simulink model "DT4V_System_Model_v17_ref_speed_R2019a"  (R2023a)
settings: Solver=ode4  StartTime=0.0  StopTime=Config.Tsim  FixedStep=Config.Ts  RelTol=1e-3
undefined symbols (not defined in the file or in its folder): CC, Config, DCL, DiscIntNeverNeededParam, EM, GB, Grid, Inv, LM, Ma_1D, Psw_1D, Rceon_1D, Rec, Vceon_1D
libraries: simulink x3, DT4V_LoadModels x2
(part 2 of 2)

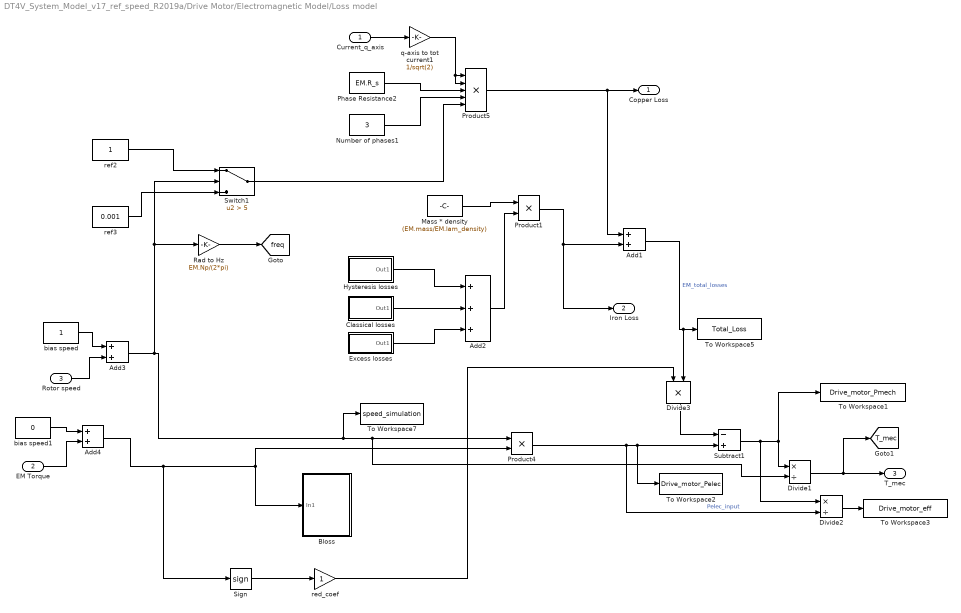
== system DT4V_System_Model_v17_ref_speed_R2019a/Drive Motor/Electromagnetic Model/Loss model ==
  Current_q_axis : Inport
  EM Torque : Inport  Port=2
  Rotor speed : Inport  Port=3
  Add1 : Sum
  Add2 : Sum  Inputs=+++
  Add3 : Sum
  Add4 : Sum
  Bloss : Subsystem
  Classical losses : Subsystem
  Divide1 : Product  Inputs=*/
  Divide2 : Product  Inputs=*/
  Divide3 : Product  Inputs=**
  Excess losses : Subsystem
  Hysteresis losses : Subsystem
  Mass * density : Constant  Value=(EM.mass/EM.lam_density)
  Number of phases1 : Constant  Value=3
  Phase Resistance2 : Constant  Value=EM.R_s
  Product1 : Product
  Product4 : Product
  Product5 : Product  Inputs=5
  Rad to Hz : Gain  Gain=EM.Np/(2*pi)
  Sign : Signum
  Subtract1 : Sum  Inputs=-+
  Switch1 : Switch  Criteria=u2 > Threshold  Threshold=5  SaturateOnIntegerOverflow=off  InputSameDT=off
  To Workspace1 : ToWorkspace  VariableName=Drive_motor_Pmech  SampleTime=-1
      settings: Save2DSignal=2-D array (concatenate along first dimension)
  To Workspace2 : ToWorkspace  VariableName=Drive_motor_Pelec  SampleTime=-1
      settings: Save2DSignal=2-D array (concatenate along first dimension)
  To Workspace3 : ToWorkspace  VariableName=Drive_motor_eff  SampleTime=-1
      settings: Save2DSignal=2-D array (concatenate along first dimension)
  To Workspace5 : ToWorkspace  VariableName=Total_Loss  SampleTime=-1
      settings: Save2DSignal=2-D array (concatenate along first dimension)
  To Workspace7 : ToWorkspace  VariableName=speed_simulation  SampleTime=-1
      settings: Save2DSignal=2-D array (concatenate along first dimension)
  bias speed : Constant
  bias speed1 : Constant  Value=0
  q-axis to tot current1 : Gain  Gain=1/sqrt(2)
  red_coef : Gain
  ref2 : Constant
  ref3 : Constant  Value=0.001
  "Copper Loss " : Outport
  Iron Loss : Outport  Port=2
  T_mec : Outport  Port=3
  tag scope: T_mec=global, freq=global
  wires:
  Product1/1 -> Iron Loss/1, Add1/2
  Number of phases1/1 -> Product5/4
  Excess losses/1(Out1) -> Add2/3
  Hysteresis losses/1(Out1) -> Add2/1
  Rad to Hz/1 -> [freq]
  Add1/1 -> To Workspace5/1, Divide3/2  "EM_total_losses"
  Subtract1/1 -> Divide2/1, Divide1/1, To Workspace1/1
  Classical losses/1(Out1) -> Add2/2
  Current_q_axis/1 -> q-axis to tot current1/1
  Phase Resistance2/1 -> Product5/3
  Add3/1 -> To Workspace7/1, Product4/1, Divide1/2, Switch1/2, Rad to Hz/1
  Product4/1 -> Divide2/2, To Workspace2/1, Subtract1/2  "Pelec_input"
  q-axis to tot current1/1 -> Product5/2, Product5/1
  Add2/1 -> Product1/2
  ref3/1 -> Switch1/3
  ref2/1 -> Switch1/1
  Divide2/1 -> To Workspace3/1
  Divide1/1 -> [T_mec], T_mec/1
  Add4/1 -> Sign/1, Product4/2, Bloss/1(In1)
  Sign/1 -> red_coef/1
  Product5/1 -> "Copper Loss "/1, Add1/1
  Divide3/1 -> Subtract1/1
  red_coef/1 -> Divide3/1
  bias speed/1 -> Add3/1
  Rotor speed/1 -> Add3/2
  Switch1/1 -> Product5/5
  bias speed1/1 -> Add4/1
  EM Torque/1 -> Add4/2
  Mass * density/1 -> Product1/1

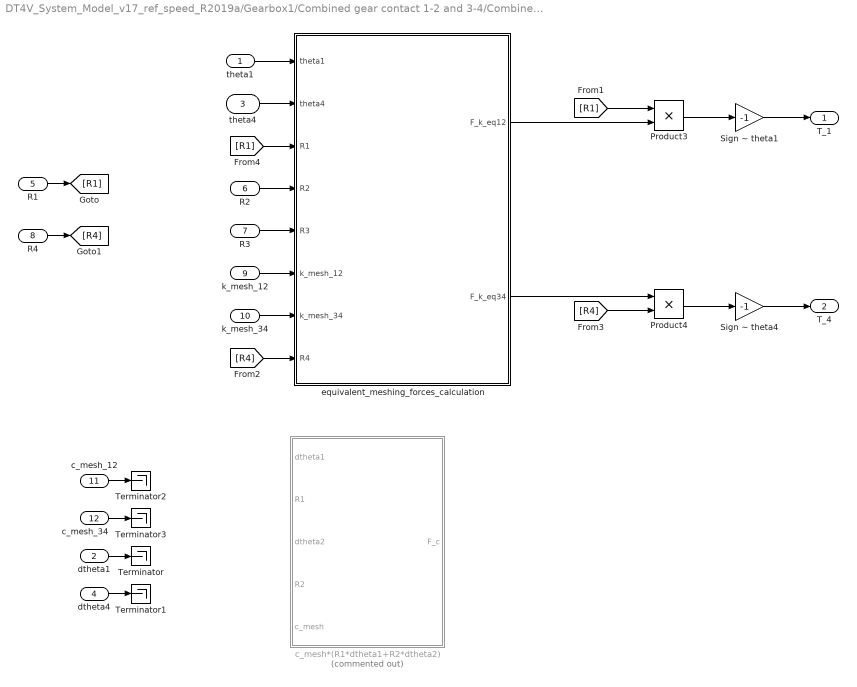
== system DT4V_System_Model_v17_ref_speed_R2019a/Gearbox1/Combined gear contact 1-2 and 3-4/Combined contact 1-2, 3-4 ==
  theta1 : Inport
  dtheta1 : Inport  Port=2
  theta4 : Inport  Port=3
  dtheta4 : Inport  Port=4
  R1 : Inport  Port=5
  R2 : Inport  Port=6
  R3 : Inport  Port=7
  R4 : Inport  Port=8
  k_mesh_12 : Inport  Port=9
  k_mesh_34 : Inport  Port=10
  c_mesh_12 : Inport  Port=11
  c_mesh_34 : Inport  Port=12
  Product3 : Product
  Product4 : Product
  Sign ~ theta1 : Gain  Gain=-1
  Sign ~ theta4 : Gain  Gain=-1
  Terminator{,1..3} (4 alike) : Terminator
  c_mesh*(R1*dtheta1+R2*dtheta2) : Subsystem  Commented=on
  equivalent_meshing_forces_calculation : Subsystem
  T_1 : Outport
  T_4 : Outport  Port=2
  wires:
  theta1/1 -> equivalent_meshing_forces_calculation/1(theta1)
  k_mesh_12/1 -> equivalent_meshing_forces_calculation/6(k_mesh_12)
  [R1] -> equivalent_meshing_forces_calculation/3(R1)
  [R1] -> Product3/1
  R2/1 -> equivalent_meshing_forces_calculation/4(R2)
  [R4] -> Product4/2
  equivalent_meshing_forces_calculation/1(F_k_eq12) -> Product3/2
  Product3/1 -> Sign ~ theta1/1
  Sign ~ theta1/1 -> T_1/1
  Product4/1 -> Sign ~ theta4/1
  Sign ~ theta4/1 -> T_4/1
  dtheta1/1 -> Terminator/1
  dtheta4/1 -> Terminator1/1
  c_mesh_12/1 -> Terminator2/1
  c_mesh_34/1 -> Terminator3/1
  theta4/1 -> equivalent_meshing_forces_calculation/2("theta4 ")
  R3/1 -> equivalent_meshing_forces_calculation/5(R3)
  k_mesh_34/1 -> equivalent_meshing_forces_calculation/7(k_mesh_34)
  R1/1 -> [R1]
  R4/1 -> [R4]
  [R4] -> equivalent_meshing_forces_calculation/8(R4)
  equivalent_meshing_forces_calculation/2(F_k_eq34) -> Product4/1

== system DT4V_System_Model_v17_ref_speed_R2019a/Gearbox1/Thermal model/Heat equation ==
  P_loss : Inport
  UA : Inport  Port=2
  T_ambient : Inport  Port=3
  -(T-T_env) : Sum  Inputs=-+
  1/(m*C_P) : Product  Inputs=*/
  Add : Sum  OutMin=[-1e6]  OutMax=[1e6]
  Constant1 : Constant
  Integrator : Integrator  InitialCondition=GB.oil.temp_0
  Product2 : Product
  dT_dt : Product
  mcp : Constant  Value=GB.thermal.mcpeq
  T : Outport
  wires:
  -(T-T_env)/1 -> Product2/2
  UA/1 -> Product2/1
  Product2/1 -> Add/2
  1/(m*C_P)/1 -> dT_dt/2
  Add/1 -> dT_dt/1
  Constant1/1 -> 1/(m*C_P)/1
  P_loss/1 -> Add/1
  T_ambient/1 -> -(T-T_env)/2
  dT_dt/1 -> Integrator/1
  Integrator/1 -> -(T-T_env)/1, T/1
  mcp/1 -> 1/(m*C_P)/2

== system DT4V_System_Model_v17_ref_speed_R2019a/Gearbox1/Zero inertia gear 1/Sign & maximum for loss term ==
  T_loss : Inport
  Speed : Inport  Port=2
  T_in : Inport  Port=3
  Abs1 : Abs  SaturateOnIntegerOverflow=off
  Abs2 : Abs  SaturateOnIntegerOverflow=off
  Gain1 : Gain  Gain=-1
  Gain2 : Gain  Gain=-1
  OR : Sum
  Relational Operator1 : RelationalOperator  Operator=<  OutDataTypeStr=boolean  RndMeth=Simplest  InputSameDT=off
  Should be positive (Just to be sure) : Abs  SaturateOnIntegerOverflow=off
  Sign loss torque : Switch  Criteria=u2 > Threshold  SaturateOnIntegerOverflow=off  InputSameDT=off
  Speed threshold : Constant  Value=0.001
  "Standard - loss opposite sign to speed Very low speed - loss opposite sign to torque " : Switch  Criteria=u2 > Threshold  SaturateOnIntegerOverflow=off  InputSameDT=off
  Very low speed Max. |T_loss| = |T_in| : Switch  Criteria=u2 > Threshold  SaturateOnIntegerOverflow=off  InputSameDT=off
  |T_loss| <= |T_in| : RelationalOperator  Operator=<=  OutDataTypeStr=boolean  RndMeth=Simplest  InputSameDT=off
  T_loss_correct_sign : Outport
  wires:
  T_in/1 -> "Standard - loss opposite sign to speed Very low speed - loss opposite sign to torque "/3, Abs1/1, Gain2/1
  Relational Operator1/1 -> "Standard - loss opposite sign to speed Very low speed - loss opposite sign to torque "/2, OR/2
  |T_loss| <= |T_in|/1 -> OR/1
  Should be positive (Just to be sure)/1 -> |T_loss| <= |T_in|/1, Sign loss torque/3, Gain1/1
  OR/1 -> Very low speed Max. |T_loss| = |T_in|/2
  Abs2/1 -> Relational Operator1/2
  Gain1/1 -> Sign loss torque/1
  Speed threshold/1 -> Relational Operator1/1
  Abs1/1 -> |T_loss| <= |T_in|/2
  Sign loss torque/1 -> Very low speed Max. |T_loss| = |T_in|/1
  Gain2/1 -> Very low speed Max. |T_loss| = |T_in|/3
  "Standard - loss opposite sign to speed Very low speed - loss opposite sign to torque "/1 -> Sign loss torque/2
  Speed/1 -> "Standard - loss opposite sign to speed Very low speed - loss opposite sign to torque "/1, Abs2/1
  Very low speed Max. |T_loss| = |T_in|/1 -> T_loss_correct_sign/1
  T_loss/1 -> Should be positive (Just to be sure)/1

== system DT4V_System_Model_v17_ref_speed_R2019a/Gearbox1/Zero inertia gear 4/Sign & maximum for loss term ==
  T_loss : Inport
  Speed : Inport  Port=2
  T_in : Inport  Port=3
  Abs1 : Abs  SaturateOnIntegerOverflow=off
  Abs2 : Abs  SaturateOnIntegerOverflow=off
  Gain1 : Gain  Gain=-1
  Gain2 : Gain  Gain=-1
  OR : Sum
  Relational Operator1 : RelationalOperator  Operator=<  OutDataTypeStr=boolean  RndMeth=Simplest  InputSameDT=off
  Should be positive (Just to be sure) : Abs  SaturateOnIntegerOverflow=off
  Sign loss torque : Switch  Criteria=u2 > Threshold  SaturateOnIntegerOverflow=off  InputSameDT=off
  Speed threshold : Constant  Value=0.001
  "Standard - loss opposite sign to speed Very low speed - loss opposite sign to torque " : Switch  Criteria=u2 > Threshold  SaturateOnIntegerOverflow=off  InputSameDT=off
  Very low speed Max. |T_loss| = |T_in| : Switch  Criteria=u2 > Threshold  SaturateOnIntegerOverflow=off  InputSameDT=off
  |T_loss| <= |T_in| : RelationalOperator  Operator=<=  OutDataTypeStr=boolean  RndMeth=Simplest  InputSameDT=off
  T_loss_correct_sign : Outport
  wires:
  T_in/1 -> "Standard - loss opposite sign to speed Very low speed - loss opposite sign to torque "/3, Abs1/1, Gain2/1
  Relational Operator1/1 -> "Standard - loss opposite sign to speed Very low speed - loss opposite sign to torque "/2, OR/2
  |T_loss| <= |T_in|/1 -> OR/1
  Should be positive (Just to be sure)/1 -> |T_loss| <= |T_in|/1, Sign loss torque/3, Gain1/1
  OR/1 -> Very low speed Max. |T_loss| = |T_in|/2
  Abs2/1 -> Relational Operator1/2
  Gain1/1 -> Sign loss torque/1
  Speed threshold/1 -> Relational Operator1/1
  Abs1/1 -> |T_loss| <= |T_in|/2
  Sign loss torque/1 -> Very low speed Max. |T_loss| = |T_in|/1
  Gain2/1 -> Very low speed Max. |T_loss| = |T_in|/3
  "Standard - loss opposite sign to speed Very low speed - loss opposite sign to torque "/1 -> Sign loss torque/2
  Speed/1 -> "Standard - loss opposite sign to speed Very low speed - loss opposite sign to torque "/1, Abs2/1
  Very low speed Max. |T_loss| = |T_in|/1 -> T_loss_correct_sign/1
  T_loss/1 -> Should be positive (Just to be sure)/1

== system DT4V_System_Model_v17_ref_speed_R2019a/Power Electronics2/AC//DC Converter/DC Bus model ==
  In1 : Inport
  1/C : Gain  Gain=1/(DCL.Cap.C_C_f)
  1/Rp : Gain  Gain=1/(DCL.Cap.Rp_C_ohm)
  Add : Sum  Inputs=+++
  Add1 : Sum  Inputs=-+
  Constant4 : Constant  Value=DCL.Cap.Vdc_C_v
  Integrator : Integrator  LimitOutput=on  UpperSaturationLimit=5  LowerSaturationLimit=-10  IgnoreLimit=on
  Memory : Memory
  Saturation : Saturate  UpperLimit=DCL.Cap.Vdcmax_C_v  LowerLimit=DCL.Cap.Vdcmin_C_v
  Transfer Fcn : TransferFcn  Denominator=[0.001 1]
  esr : Gain  Gain=DCL.Cap.ESR_C_ohm
  Voltage_DC_bus : Outport
  wires:
  In1/1 -> Transfer Fcn/1  "IDC_bus"
  Add/1 -> Saturation/1
  Constant4/1 -> Add/3
  Saturation/1 -> Voltage_DC_bus/1
  Add1/1 -> Memory/1, 1/C/1  "ic"
  1/C/1 -> Integrator/1
  Memory/1 -> 1/Rp/1
  Integrator/1 -> Add/1
  Transfer Fcn/1 -> Add1/2, esr/1
  esr/1 -> Add/2
  1/Rp/1 -> Add1/1

== system DT4V_System_Model_v17_ref_speed_R2019a/Power Electronics2/AC//DC Converter/Half-Bridge 1  ==
  Vdc : Inport
  Iphase : Inport  Port=2
  Constant4 : Constant  Value=Rec.Di.R0_3D_ohm
  Constant5 : Constant  Value=Rec.Di.VT_3D_v
  MATLAB Function : MATLAB Function  TreatAsAtomicUnit=on
  Vphase : Outport
  Idc : Outport  Port=2
  DiodeLosses1Phase : Outport  Port=3
  wires:
  Vdc/1 -> MATLAB Function/1(Vdc)
  MATLAB Function/2(Idc) -> Idc/1
  MATLAB Function/3(Pcond) -> DiodeLosses1Phase/1
  Iphase/1 -> MATLAB Function/2(Iphase)
  MATLAB Function/1(Vphase) -> Vphase/1
  Constant5/1 -> MATLAB Function/3(VT)
  Constant4/1 -> MATLAB Function/4(R_0)

== system DT4V_System_Model_v17_ref_speed_R2019a/Power Electronics2/AC//DC Converter/Half-Bridge 2 ==
  Vdc : Inport
  Iphase : Inport  Port=2
  Constant4 : Constant  Value=Rec.Di.R0_3D_ohm
  Constant5 : Constant  Value=Rec.Di.VT_3D_v
  MATLAB Function : MATLAB Function  TreatAsAtomicUnit=on
  Vphase : Outport
  Idc : Outport  Port=2
  DiodeLosses1Phase : Outport  Port=3
  wires:
  Vdc/1 -> MATLAB Function/1(Vdc)
  Iphase/1 -> MATLAB Function/2(Iphase)
  MATLAB Function/3(Pcond) -> DiodeLosses1Phase/1
  MATLAB Function/1(Vphase) -> Vphase/1
  MATLAB Function/2(Idc) -> Idc/1
  Constant4/1 -> MATLAB Function/4(R_0)
  Constant5/1 -> MATLAB Function/3(VT)

== system DT4V_System_Model_v17_ref_speed_R2019a/Power Electronics2/AC//DC Converter/Half-Bridge 3 ==
  Vdc : Inport
  Iphase : Inport  Port=2
  Constant4 : Constant  Value=Rec.Di.R0_3D_ohm
  Constant5 : Constant  Value=Rec.Di.VT_3D_v
  MATLAB Function : MATLAB Function  TreatAsAtomicUnit=on
  Vphase : Outport
  Idc : Outport  Port=2
  DiodeLosses1Phase : Outport  Port=3
  wires:
  Vdc/1 -> MATLAB Function/1(Vdc)
  Iphase/1 -> MATLAB Function/2(Iphase)
  MATLAB Function/3(Pcond) -> DiodeLosses1Phase/1
  MATLAB Function/1(Vphase) -> Vphase/1
  MATLAB Function/2(Idc) -> Idc/1
  Constant4/1 -> MATLAB Function/4(R_0)
  Constant5/1 -> MATLAB Function/3(VT)

== system DT4V_System_Model_v17_ref_speed_R2019a/Power Electronics2/AC//DC Converter/OverVoltage Control Block ==
  Enable/Disable : Inport
  Idc : Inport  Port=2
  AND : Logic  AllPortsSameDT=off  OutDataTypeStr=boolean
  Compare To Constant10 : simulink/Logic and Bit Operations/Compare To Constant  relop=<=  const=1  OutDataTypeStr=boolean
  Constant : Constant  Value=0
  Constant1 : Constant  Value=10
  Initial condition : Switch  Criteria=u2 > Threshold  SaturateOnIntegerOverflow=off  InputSameDT=off
  Memory : Memory
  Moving RMS Calculation Triggered Subsystem : Subsystem  TreatAsAtomicUnit=on
  Pulse Generator2 : DiscretePulseGenerator  PulseType=Time based  Period=Config.MovingRMS.Time  PulseWidth=((Config.MovingRMS.Time-Config.Ts)/(Config.MovingRMS.Time))*100  VectorParams1D=off
  Rate Transition : RateTransition  Deterministic=off  OutPortSampleTimeMultiple=Config.MovingRMS.Time  OutPortSampleTime=Config.MovingRMS.Time
  Step : Step  Time=Config.MovingRMS.Time  Before=1  After=0  SampleTime=0
  Switch : Switch  Criteria=u2 > Threshold  SaturateOnIntegerOverflow=off  InputSameDT=off
  Out1 : Outport
  wires:
  Switch/1 -> Out1/1
  AND/1 -> Switch/2
  Idc/1 -> Switch/3, Moving RMS Calculation Triggered Subsystem/1(In1)
  Pulse Generator2/1 -> Moving RMS Calculation Triggered Subsystem/Enable
  Constant/1 -> Switch/1
  Moving RMS Calculation Triggered Subsystem/1(Out1) -> Memory/1
  Step/1 -> Initial condition/2
  Rate Transition/1 -> Initial condition/3
  Constant1/1 -> Initial condition/1
  Memory/1 -> Rate Transition/1
  Initial condition/1 -> Compare To Constant10/1
  Enable/Disable/1 -> AND/2
  Compare To Constant10/1 -> AND/1

== system DT4V_System_Model_v17_ref_speed_R2019a/Power Electronics2/DC//AC Converter/AC Ouput power measurment ==
  Current : Inport
  Voltage : Inport  Port=2
  Product1 : Product  InputSameDT=on  SaturateOnIntegerOverflow=on  OutDataTypeStr=Inherit: Same as first input
  Sum4 : Sum  Inputs=1  InputSameDT=on  SaturateOnIntegerOverflow=on  OutDataTypeStr=Inherit: Same as first input
  Transfer Fcn1 : TransferFcn  Denominator=[0.005 1]
  AC ouput power : Outport
  wires:
  Voltage/1 -> Product1/2
  Current/1 -> Product1/1
  Product1/1 -> Sum4/1
  Sum4/1 -> Transfer Fcn1/1  "P"
  Transfer Fcn1/1 -> AC ouput power/1

== system DT4V_System_Model_v17_ref_speed_R2019a/Power Electronics2/DC//AC Converter/DC Input power measurment ==
  Current : Inport
  Voltage : Inport  Port=2
  Product1 : Product  InputSameDT=on  SaturateOnIntegerOverflow=on  OutDataTypeStr=Inherit: Same as first input
  Transfer Fcn1 : TransferFcn  Denominator=[0.005 1]
  DC input power : Outport
  wires:
  Product1/1 -> Transfer Fcn1/1  "P"
  Current/1 -> Product1/1
  Voltage/1 -> Product1/2
  Transfer Fcn1/1 -> DC input power/1

== system DT4V_System_Model_v17_ref_speed_R2019a/Power Electronics2/DC//AC Converter/Half-Bridge 1 ==
  d : Inport
  Vdc : Inport  Port=2
  Iphase : Inport  Port=3
  Constant2 : Constant  Value=Inv.IGBT.Rce_3D_ohm
  Constant3 : Constant  Value=Inv.IGBT.Vce_3D_v
  Constant4 : Constant  Value=Inv.Di.Rd_3D_ohm
  Constant5 : Constant  Value=Inv.Di.Vf_3D_v
  MATLAB Function : MATLAB Function  TreatAsAtomicUnit=on
  Vphase : Outport
  Idc : Outport  Port=2
  tag scope: P_cond_1=global
  wires:
  d/1 -> MATLAB Function/1(d)
  Vdc/1 -> MATLAB Function/2(Vdc)
  Iphase/1 -> MATLAB Function/3(Iphase)
  Constant2/1 -> MATLAB Function/5(Rce_on)
  Constant4/1 -> MATLAB Function/7(Rd)
  Constant3/1 -> MATLAB Function/4(Vce_on)
  Constant5/1 -> MATLAB Function/6(Vf_0)
  MATLAB Function/1(Vphase) -> Vphase/1
  MATLAB Function/2(Idc) -> Idc/1
  MATLAB Function/3(Pcond) -> [P_cond_1]

== system DT4V_System_Model_v17_ref_speed_R2019a/Power Electronics2/DC//AC Converter/Half-Bridge 2 ==
  d : Inport
  Vdc : Inport  Port=2
  Iphase : Inport  Port=3
  Constant2 : Constant  Value=Inv.IGBT.Rce_3D_ohm
  Constant3 : Constant  Value=Inv.IGBT.Vce_3D_v
  Constant4 : Constant  Value=Inv.Di.Rd_3D_ohm
  Constant5 : Constant  Value=Inv.Di.Vf_3D_v
  MATLAB Function : MATLAB Function  TreatAsAtomicUnit=on
  Vphase : Outport
  Idc : Outport  Port=2
  tag scope: P_cond_2=global
  wires:
  MATLAB Function/3(Pcond) -> [P_cond_2]
  MATLAB Function/1(Vphase) -> Vphase/1
  d/1 -> MATLAB Function/1(d)
  Iphase/1 -> MATLAB Function/3(Iphase)
  Constant4/1 -> MATLAB Function/7(Rd)
  Constant3/1 -> MATLAB Function/4(Vce_on)
  Constant2/1 -> MATLAB Function/5(Rce_on)
  Vdc/1 -> MATLAB Function/2(Vdc)
  Constant5/1 -> MATLAB Function/6(Vf_0)
  MATLAB Function/2(Idc) -> Idc/1

== system DT4V_System_Model_v17_ref_speed_R2019a/Power Electronics2/DC//AC Converter/Half-Bridge 3 ==
  d : Inport
  Vdc : Inport  Port=2
  Iphase : Inport  Port=3
  Constant2 : Constant  Value=Inv.IGBT.Rce_3D_ohm
  Constant3 : Constant  Value=Inv.IGBT.Vce_3D_v
  Constant4 : Constant  Value=Inv.Di.Rd_3D_ohm
  Constant5 : Constant  Value=Inv.Di.Vf_3D_v
  MATLAB Function : MATLAB Function  TreatAsAtomicUnit=on
  Vphase : Outport
  Idc : Outport  Port=2
  tag scope: P_cond_3=global
  wires:
  MATLAB Function/3(Pcond) -> [P_cond_3]
  MATLAB Function/1(Vphase) -> Vphase/1
  d/1 -> MATLAB Function/1(d)
  Iphase/1 -> MATLAB Function/3(Iphase)
  Constant4/1 -> MATLAB Function/7(Rd)
  Constant3/1 -> MATLAB Function/4(Vce_on)
  Constant2/1 -> MATLAB Function/5(Rce_on)
  Vdc/1 -> MATLAB Function/2(Vdc)
  Constant5/1 -> MATLAB Function/6(Vf_0)
  MATLAB Function/2(Idc) -> Idc/1

== system DT4V_System_Model_v17_ref_speed_R2019a/Power Electronics2/DC//AC Converter/Loss Model ==
  speed : Inport
  Torque : Inport  Port=2
  Power_Loss_Model1 : Subsystem  mask{sfcnParam1=Ma_1D, sfcnParam2=Psw_1D, sfcnParam3=Rceon_1D, sfcnParam4=Vceon_1D}
      mask prompts: sfcnParam1 "Ma_1D:"; sfcnParam2 "Psw_1D:"; sfcnParam3 "Rceon_1D:"; sfcnParam4 "Vceon_1D:"
      mask help: Simulink:masks:GenSFuncDesc_MD
      mask Help: eval('feval(''rtwprivate'',''rtwhelpview'',''rtw_sfcn_block'')');
  Sum3 : Sum  Inputs=+++
  Sum6 : Sum  Inputs=-+
  Transfer Fcn1 : TransferFcn  Denominator=[0.005 1]
  Transfer Fcn2 : TransferFcn  Denominator=[0.005 1]
  Inverter_total_loss : Outport
  tag scope: P_d=global
  wires:
  Transfer Fcn2/1 -> Inverter_total_loss/1
  Torque/1 -> Power_Loss_Model1/2(Torque)
  Power_Loss_Model1/1(Estimated loss) -> Transfer Fcn2/1, Sum6/2
  Sum3/1 -> Sum6/1
  speed/1 -> Power_Loss_Model1/1(speed)
  Transfer Fcn1/1 -> [P_d]
  [P_cond_3] -> Sum3/3
  [P_cond_1] -> Sum3/1
  Sum6/1 -> Transfer Fcn1/1  "LOSS model"
  [P_cond_2] -> Sum3/2

== system DT4V_System_Model_v17_ref_speed_R2019a/Power Electronics2/DC//AC Converter/Subsystem ==
  Compare To Constant : simulink/Logic and Bit Operations/Compare To Constant  relop=<=  const=-10  OutDataTypeStr=boolean
  Compare To Constant1 : simulink/Logic and Bit Operations/Compare To Constant  relop=>=  const=10  OutDataTypeStr=boolean
  Constant2 : Constant  Value=inf
  Divide1 : Product  Inputs=*/
  OR : Logic  Operator=OR  IconShape=distinctive  AllPortsSameDT=off  OutDataTypeStr=boolean
  Saturation : Saturate  UpperLimit=inf  LowerLimit=0
  Switch : Switch  Criteria=u2 > Threshold  SaturateOnIntegerOverflow=off  InputSameDT=off
  Idc2 : Outport
  wires:
  Constant2/1 -> Switch/3
  Switch/1 -> Divide1/2
  Compare To Constant1/1 -> OR/1
  [P_d] -> Divide1/1
  Compare To Constant/1 -> OR/2
  OR/1 -> Switch/2
  Divide1/1 -> Saturation/1
  Saturation/1 -> Idc2/1
  [AC_POWER] -> Compare To Constant/1, Compare To Constant1/1, Switch/1

== system DT4V_System_Model_v17_ref_speed_R2019a/Drive Motor/Electromagnetic Model/Electromagnetic model/Stator flux calculation ==
  "Iq " : Inport
  Id1 : Inport  Port=2
  Add : Sum
  L_d2 : Gain  Gain=EM.L_d
  L_q1 : Gain  Gain=EM.L_q
  MATLAB Function : MATLAB Function  TreatAsAtomicUnit=on
  Scope : Scope
  To Workspace : ToWorkspace  VariableName=Psi  SaveFormat=Timeseries  SampleTime=-1
  To Workspace1 : ToWorkspace  VariableName=PsiTs  SaveFormat=Timeseries  SampleTime=-1
  Zero-Order Hold : ZeroOrderHold  SampleTime=-1
  i_mag1 : Constant  Value=EM.i_mag
  wires:
  "Iq "/1 -> L_q1/1
  Id1/1 -> Add/1
  i_mag1/1 -> Add/2
  Add/1 -> L_d2/1
  L_q1/1 -> MATLAB Function/1(Psi_q_2)
  L_d2/1 -> MATLAB Function/2(Psi_d_2)
  MATLAB Function/1(Psi_tot) -> Zero-Order Hold/1, To Workspace/1, Scope/1
  Zero-Order Hold/1 -> To Workspace1/1

== system DT4V_System_Model_v17_ref_speed_R2019a/Drive Motor/Electromagnetic Model/Loss model/Bloss ==
  In1 : Inport
  " Bmax" : Constant  Value=EM.Bmax
  " xfactor" : Constant  Value=EM.xfactor
  Abs1 : Abs  SaturateOnIntegerOverflow=off
  Add2 : Sum
  Product1 : Product
  rated_torque : Gain  Gain=1/EM.torque
  tag scope: Bloss=global
  wires:
  Add2/1 -> [Bloss]
  In1/1 -> Abs1/1
  rated_torque/1 -> Product1/2
  " Bmax"/1 -> Add2/1
  " xfactor"/1 -> Product1/1
  Product1/1 -> Add2/2  "Pelec_input"
  Abs1/1 -> rated_torque/1

== system DT4V_System_Model_v17_ref_speed_R2019a/Drive Motor/Electromagnetic Model/Loss model/Classical losses ==
  "   " : Constant  Value=EM.alfa2
  "Classical " : Gain  Gain=EM.k2
  Power : Math  Operator=pow  SignedPower=on
  Power3 : Math  Operator=pow  SignedPower=on
  Product4 : Product
  alfa2 : Constant  Value=EM.alfa2
  Out1 : Outport
  wires:
  Power/1 -> Product4/1
  alfa2/1 -> Power/2
  Product4/1 -> "Classical "/1
  Power3/1 -> Product4/2
  [freq] -> Power/1
  "Classical "/1 -> Out1/1
  [Bloss] -> Power3/1
  "   "/1 -> Power3/2

== system DT4V_System_Model_v17_ref_speed_R2019a/Drive Motor/Electromagnetic Model/Loss model/Excess losses ==
  " " : Constant  Value=1.5
  "  " : Constant  Value=1.5
  Excess : Gain  Gain=EM.k3
  Power1 : Math  Operator=pow  SignedPower=on
  Power3 : Math  Operator=pow  SignedPower=on
  Product4 : Product
  Out1 : Outport
  wires:
  Product4/1 -> Excess/1
  " "/1 -> Power1/2
  "  "/1 -> Power3/2
  [freq] -> Power1/1
  Power1/1 -> Product4/1
  [Bloss] -> Power3/1
  Excess/1 -> Out1/1
  Power3/1 -> Product4/2

== system DT4V_System_Model_v17_ref_speed_R2019a/Drive Motor/Electromagnetic Model/Loss model/Hysteresis losses ==
  "  " : Constant  Value=EM.alfa1
  Hysteresis : Gain  Gain=EM.k1
  Power2 : Math  Operator=pow  SignedPower=on
  Product1 : Product
  Out1 : Outport
  wires:
  "  "/1 -> Power2/2
  [freq] -> Product1/1
  Power2/1 -> Product1/2
  Product1/1 -> Hysteresis/1
  Hysteresis/1 -> Out1/1
  [Bloss] -> Power2/1

== system DT4V_System_Model_v17_ref_speed_R2019a/Gearbox1/Combined gear contact 1-2 and 3-4/Combined contact 1-2, 3-4/c_mesh*(R1*dtheta1+R2*dtheta2) ==
  dtheta1 : Inport
  R1 : Inport  Port=2
  dtheta2 : Inport  Port=3
  R2 : Inport  Port=4
  c_mesh : Inport  Port=5
  Add : Sum
  Product : Product
  Product1 : Product
  Product2 : Product
  F_c : Outport
  wires:
  R2/1 -> Product1/2
  Product1/1 -> Add/2
  Product/1 -> Add/1
  dtheta2/1 -> Product1/1
  Add/1 -> Product2/1
  c_mesh/1 -> Product2/2
  Product2/1 -> F_c/1
  dtheta1/1 -> Product/1
  R1/1 -> Product/2

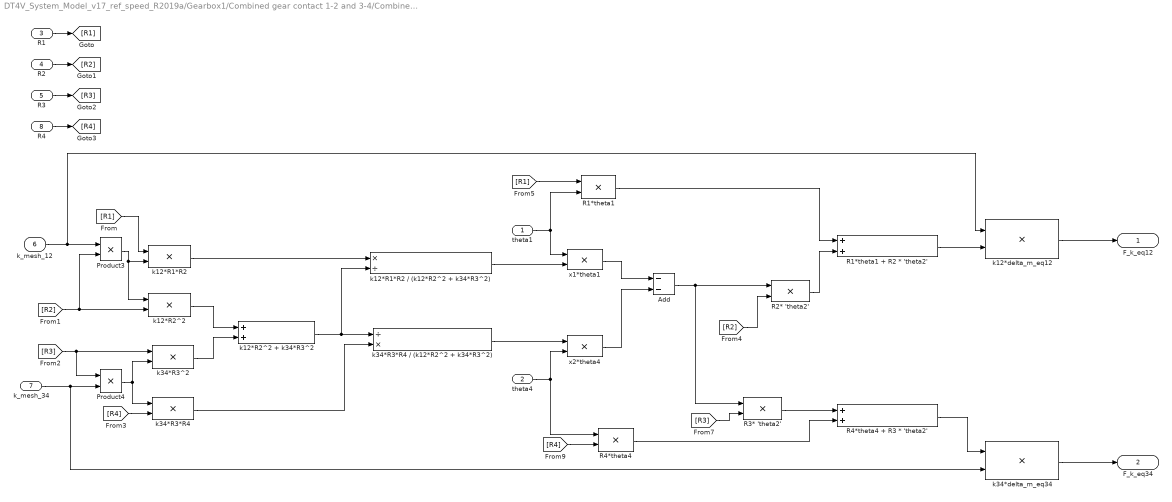
== system DT4V_System_Model_v17_ref_speed_R2019a/Gearbox1/Combined gear contact 1-2 and 3-4/Combined contact 1-2, 3-4/equivalent_meshing_forces_calculation ==
  theta1 : Inport
  "theta4 " : Inport  Port=2
  R1 : Inport  Port=3
  R2 : Inport  Port=4
  R3 : Inport  Port=5
  k_mesh_12 : Inport  Port=6
  k_mesh_34 : Inport  Port=7
  R4 : Inport  Port=8
  Add : Sum  Inputs=--
  Product3 : Product
  Product4 : Product
  R1*theta1 : Product
  R1*theta1 + R2 * 'theta2' : Sum
  R2* 'theta2' : Product
  R3* 'theta2' : Product
  R4*theta4 : Product
  R4*theta4 + R3 * 'theta2' : Sum
  k12*R1*R2 : Product
  k12*R1*R2 / (k12*R2^2 + k34*R3^2) : Product  Inputs=*/
  k12*R2^2 : Product
  k12*R2^2 + k34*R3^2 : Sum
  k12*delta_m_eq12 : Product
  k34*R3*R4 : Product
  k34*R3*R4 / (k12*R2^2 + k34*R3^2) : Product  Inputs=/*
  k34*R3^2 : Product
  k34*delta_m_eq34 : Product
  x1*theta1 : Product
  x2*theta4 : Product
  F_k_eq12 : Outport
  F_k_eq34 : Outport  Port=2
  wires:
  x2*theta4/1 -> Add/2
  x1*theta1/1 -> Add/1
  Add/1 -> R3* 'theta2'/1, R2* 'theta2'/1
  k_mesh_12/1 -> k12*delta_m_eq12/1, Product3/1
  Product3/1 -> k12*R2^2/1, k12*R1*R2/2
  Product4/1 -> k34*R3*R4/1, k34*R3^2/2
  k12*R2^2/1 -> k12*R2^2 + k34*R3^2/1
  k34*R3^2/1 -> k12*R2^2 + k34*R3^2/2
  k_mesh_34/1 -> k34*delta_m_eq34/2, Product4/2
  k12*R2^2 + k34*R3^2/1 -> k34*R3*R4 / (k12*R2^2 + k34*R3^2)/1, k12*R1*R2 / (k12*R2^2 + k34*R3^2)/2
  k12*R1*R2/1 -> k12*R1*R2 / (k12*R2^2 + k34*R3^2)/1
  k34*R3*R4/1 -> k34*R3*R4 / (k12*R2^2 + k34*R3^2)/2
  R1/1 -> [R1]
  [R1] -> k12*R1*R2/1
  [R2] -> Product3/2, k12*R2^2/2
  R2/1 -> [R2]
  [R3] -> Product4/1, k34*R3^2/1
  R3/1 -> [R3]
  R4/1 -> [R4]
  [R4] -> k34*R3*R4/2
  "theta4 "/1 -> x2*theta4/2, R4*theta4/1
  theta1/1 -> R1*theta1/2, x1*theta1/1
  k34*R3*R4 / (k12*R2^2 + k34*R3^2)/1 -> x2*theta4/1
  k12*R1*R2 / (k12*R2^2 + k34*R3^2)/1 -> x1*theta1/2
  [R2] -> R2* 'theta2'/2
  [R1] -> R1*theta1/1
  R1*theta1/1 -> R1*theta1 + R2 * 'theta2'/1
  R2* 'theta2'/1 -> R1*theta1 + R2 * 'theta2'/2
  k12*delta_m_eq12/1 -> F_k_eq12/1
  k34*delta_m_eq34/1 -> F_k_eq34/1
  [R3] -> R3* 'theta2'/2
  R4*theta4 + R3 * 'theta2'/1 -> k34*delta_m_eq34/1
  R3* 'theta2'/1 -> R4*theta4 + R3 * 'theta2'/1
  [R4] -> R4*theta4/2
  R4*theta4/1 -> R4*theta4 + R3 * 'theta2'/2
  R1*theta1 + R2 * 'theta2'/1 -> k12*delta_m_eq12/2

== system DT4V_System_Model_v17_ref_speed_R2019a/Power Electronics2/AC//DC Converter/OverVoltage Control Block/Moving RMS Calculation Triggered Subsystem ==
  In1 : Inport
  Enable : EnablePort  StatesWhenEnabling=reset  PropagateVarSize=During execution
  Add : Sum
  Constant : Constant  Value=Config.MovingRMS.Time/Config.Ts
  Divide : Product  Inputs=**
  Divide1 : Product  Inputs=*/
  Memory : Memory
  Square Root : Sqrt
  Out1 : Outport
  wires:
  Divide1/1 -> Square Root/1
  Constant/1 -> Divide1/2
  Memory/1 -> Add/1
  Add/1 -> Memory/1, Divide1/1
  Divide/1 -> Add/2
  In1/1 -> Divide/1, Divide/2
  Square Root/1 -> Out1/1

== system DT4V_System_Model_v17_ref_speed_R2019a/Power Electronics2/DC//AC Converter/Loss Model/Power_Loss_Model1 ==
  speed : Inport
  Torque : Inport  Port=2
  Power_Loss_Model_sfcn : S-Function  FunctionName=Power_Loss_Model_sf  Parameters=sfcnParam1, sfcnParam2, sfcnParam3, sfcnParam4  SFunctionModules=""  SFunctionDeploymentMode=off  EnableBusSupport=off  mask{rtw_sf_name=Power_Loss_Model_sf, showVar=off, sfcnParam1=sfcnParam1, sfcnParam2=sfcnParam2, sfcnParam3=sfcnParam3, sfcnParam4=sfcnParam4}
      mask prompts: rtw_sf_name "Simulink:masks:GenSFuncName_MP"; showVar "Simulink:masks:GenSFuncShowModuleList_MP"; sfcnParam1 "Ma_1D:"; sfcnParam2 "Psw_1D:"; sfcnParam3 "Rceon_1D:"; sfcnParam4 "Vceon_1D:"
      mask help: Simulink:masks:GenSFuncDesc_MD
      mask init:
      | displist = '';
      | if ~strcmp(get_param(gcb, 'FunctionName'), rtw_sf_name);
      |   set_param(gcb, 'FunctionName', rtw_sf_name);
      | end
      | % Check if we are generating code
      | rtw_mode = false;
      | if strcmpi(get_param(bdroot(gcb),'SimulationStatus'),'Initializing')
      | 	rtw_mode = strcmpi(get_param(bdroot(gcb),'BuildingRTWCode'),'on') && ...
      | 		~strcmpi(get_param(bdroot(gcb),'TargetStyle'),'SimulationTarget');
      | end
      | if showVar || rtw_mode
      | 	if exist('rtwsfunc') == 2 | exist('rtwsfunc') == 6
      | 		tmplist = rtwsfunc(rtw_sf_name,gcb);
      | 		tmplist = DAStudio.message('Simulink:masks:GenSFuncListOfModules_IC', tmplist);
      | 	elseif showVar
      | 		tmplist1 = DAStudio.message('Simulink:masks:GenSFuncListOfModules_IC', '');
      |         tmplist2 = DAStudio.message('Simulink:masks:GenSFuncNotLicensed_IC');
      |         tmplist = [tmplist1 tmplist2];
      |  	end
      | end
      | if showVar
      |   displist = tmplist;
      | end
      settings: CopyFcn=|
      | if ~strcmp(get_param(gcb,'Linkstatus'),'none') && ...
      | ~strcmp(get_param(gcb,'Linkstatus'),'implicit')
      |   set_param(gcb,'LinkStatus','none');
      | end
      mask Help: eval('feval(''rtwprivate'',''rtwhelpview'',''rtw_sfcn_block'')');
      mask Display:
      | port_label('input',1,'speed');
      | port_label('input',2,'Torque');
      | port_label('output',1,'Estimated loss');
  __InputSSForSFun__ : Subsystem
  __OutputSSForSFun__ : Subsystem
  Estimated loss : Outport
  wires:
  speed/1 -> __InputSSForSFun__/1(speed)
  Torque/1 -> __InputSSForSFun__/2(Torque)
  __InputSSForSFun__/1(__UniqueOutportName__1__) -> Power_Loss_Model_sfcn/1
  __InputSSForSFun__/2(__UniqueOutportName__2__) -> Power_Loss_Model_sfcn/2
  Power_Loss_Model_sfcn/1 -> __OutputSSForSFun__/1(__UniqueInportName__1__)
  __OutputSSForSFun__/1(Estimated loss) -> Estimated loss/1

== system DT4V_System_Model_v17_ref_speed_R2019a/Power Electronics2/DC//AC Converter/Loss Model/Power_Loss_Model1/__InputSSForSFun__ ==
  speed : Inport
  Torque : Inport  Port=2
  __UniqueOutportName__1__ : Outport
  __UniqueOutportName__2__ : Outport  Port=2
  wires:
  speed/1 -> __UniqueOutportName__1__/1
  Torque/1 -> __UniqueOutportName__2__/1

== system DT4V_System_Model_v17_ref_speed_R2019a/Power Electronics2/DC//AC Converter/Loss Model/Power_Loss_Model1/__OutputSSForSFun__ ==
  __UniqueInportName__1__ : Inport
  Estimated loss : Outport
  wires:
  __UniqueInportName__1__/1 -> Estimated loss/1

== matlab function DT4V_System_Model_v17_ref_speed_R2019a/Gearbox1/Thermal model/MATLAB Function ==
  data: w input; hAEq output; TSump input; TAmb input
function hAEq = fcn(w, TSump, TAmb)

dT=TSump-TAmb;

p00=67.9782;
p10=-58.7751;
p01=27.9418;
p20=28.8784;
p11=-16.8035;
p02=-4.1414;
p30=14.2210;
p21=-3.7255;
p12=6.0689;
p40=-16.8580;
p31=8.8489;
p22=0.6417;
p50=3.5853;
p41=-1.9001;
p32=-2.6730;

dTmean=13; 
dTstd=6.957;
wmean=3000;
wstd=1183;

dT=(dT-dTmean)/dTstd;
w0=w;
w=(w-wmean)/wstd;
hAEq=p00 + p10*dT + p01*w + p20*dT^2 + p11*dT*w + p02*w^2 + p30*dT^3 + p21*dT^2*w + p12*dT*w^2 + p40*dT^4 + p31*dT^3*w + p22*dT^2*w^2 + p50*dT^5 + p41*dT^4*w + p32*dT^3*w^2;

if w0<1000 || dT>40
    wmean=4000;
    wstd=1183;
    wA=(1000-wmean)/wstd;
    wB=(1200-wmean)/wstd;
    dT=1.1485;
    
    hAEqA=p00 + p10*dT + p01*wA + p20*dT^2 + p11*dT*wA + p02*wA^2 + p30*dT^3 + p21*dT^2*wA + p12*dT*wA^2 + p40*dT^4 + p31*dT^3*wA + p22*dT^2*wA^2 + p50*dT^5 + p41*dT^4*wA + p32*dT^3*wA^2;
    hAEqB=p00 + p10*dT + p01*wB + p20*dT^2 + p11*dT*wB + p02*wB^2 + p30*dT^3 + p21*dT^2*wB + p12*dT*wB^2 + p40*dT^4 + p31*dT^3*wB + p22*dT^2*wB^2 + p50*dT^5 + p41*dT^4*wB + p32*dT^3*wB^2;

    hAEq=(hAEqB-hAEqA)/(wB-wA)*(w-wA)+hAEqA;
end
hAEq=abs(hAEq);

== matlab function DT4V_System_Model_v17_ref_speed_R2019a/Power Electronics2/DC//AC Converter/Half-Bridge 2/MATLAB Function ==
  data: d input; Vdc input; Vphase output; Iphase input; Vce_on input; Rce_on input; Vf_0 input; Rd input; Idc output; Pcond output
function [Vphase, Idc, Pcond] = fcn(d, Vdc,Iphase,  Vce_on, Rce_on,Vf_0,Rd)
td=0;
fs=0;
if d>0 
    theta_u= d-td*fs;
    theta_l=1-d-td*fs;
else
    theta_u= 0;
    theta_l=0;
end
%%%%%%%%%%%%%%%%%%%%%%

if Iphase>0 % current from brigde to motor
    Vphase= theta_u*(Vdc-(Vce_on+Rce_on*Iphase))-(1-theta_u)*(Vf_0+Rd*Iphase);
    Idc=theta_u*Iphase;
    Pcond_s1=theta_u*(Vce_on+Rce_on*Iphase)*Iphase ;
    Pcond_s2=0 ;
    Pcond_d1= 0;
    Pcond_d2= (1-theta_u)*(Vf_0+Rd*Iphase)*Iphase;
    
else
    Vphase= theta_l*(Vce_on-Rce_on*Iphase)+(1-theta_l)*(Vdc+Vf_0-Rd*Iphase);
    Idc=(1-theta_l)*Iphase;    
    Pcond_s1=0 ;
    Pcond_s2=-theta_l*(Vce_on-Rce_on*Iphase)*Iphase;
    Pcond_d1= -(1-theta_l)*(Vf_0-Rd*Iphase)*Iphase;    
    Pcond_d2= 0;
    
end
Pcond = abs(Pcond_s1)+abs(Pcond_s2)+abs(Pcond_d1)+abs(Pcond_d2);

== matlab function DT4V_System_Model_v17_ref_speed_R2019a/Power Electronics2/DC//AC Converter/Half-Bridge 3/MATLAB Function ==
  data: d input; Vdc input; Vphase output; Iphase input; Vce_on input; Rce_on input; Vf_0 input; Rd input; Idc output; Pcond output
function [Vphase, Idc, Pcond] = fcn(d, Vdc,Iphase,  Vce_on, Rce_on,Vf_0,Rd)
td=0;
fs=0;
if d>0 
    theta_u= d-td*fs;
    theta_l=1-d-td*fs;
else
    theta_u= 0;
    theta_l=0;
end
%%%%%%%%%%%%%%%%%%%%%%

if Iphase>0 % current from brigde to motor
    Vphase= theta_u*(Vdc-(Vce_on+Rce_on*Iphase))-(1-theta_u)*(Vf_0+Rd*Iphase);
    Idc=theta_u*Iphase;
    Pcond_s1=theta_u*(Vce_on+Rce_on*Iphase)*Iphase ;
    Pcond_s2=0 ;
    Pcond_d1= 0;
    Pcond_d2= (1-theta_u)*(Vf_0+Rd*Iphase)*Iphase;
    
else
    Vphase= theta_l*(Vce_on-Rce_on*Iphase)+(1-theta_l)*(Vdc+Vf_0-Rd*Iphase);
    Idc=(1-theta_l)*Iphase;    
    Pcond_s1=0 ;
    Pcond_s2=-theta_l*(Vce_on-Rce_on*Iphase)*Iphase;
    Pcond_d1= -(1-theta_l)*(Vf_0-Rd*Iphase)*Iphase;    
    Pcond_d2= 0;
    
end
Pcond = abs(Pcond_s1)+abs(Pcond_s2)+abs(Pcond_d1)+abs(Pcond_d2);

== matlab function DT4V_System_Model_v17_ref_speed_R2019a/Power Electronics2/AC//DC Converter/Half-Bridge 1 /MATLAB Function ==
  data: Vdc input; Vphase output; Iphase input; VT input; R_0 input; Idc output; Pcond output
function [Vphase, Idc, Pcond] = fcn(Vdc,Iphase,VT,R_0)


%%%%%%%%%%%%%%%%%%%%%%

if Iphase>=0 %&& Vphase1>=0.7 % current from brigde to motor
    Vphase= Vdc+VT+R_0*Iphase;
    Idc=Iphase;
    Pcond_d1= 0;
    Pcond_d2= (VT+R_0*Iphase)*Iphase;
    
else
    Vphase=-VT+R_0*Iphase;
    Idc=0;    
    Pcond_d2= 0;
    Pcond_d1= (-VT+R_0*Iphase)*Iphase;
    
end
Pcond = Pcond_d1+Pcond_d2;

== matlab function DT4V_System_Model_v17_ref_speed_R2019a/Power Electronics2/AC//DC Converter/Half-Bridge 2/MATLAB Function ==
  data: Vdc input; Vphase output; Iphase input; VT input; R_0 input; Idc output; Pcond output
function [Vphase, Idc, Pcond] = fcn(Vdc,Iphase,VT,R_0)


%%%%%%%%%%%%%%%%%%%%%%

if Iphase>=0 %&& Vphase1>=0.7 % current from brigde to motor
    Vphase= Vdc+VT+R_0*Iphase;
    Idc=Iphase;
    Pcond_d1= 0;
    Pcond_d2= (VT+R_0*Iphase)*Iphase;
    
else
    Vphase=-VT+R_0*Iphase;
    Idc=0;    
    Pcond_d2= 0;
    Pcond_d1= (-VT+R_0*Iphase)*Iphase;
    
end
Pcond = Pcond_d1+Pcond_d2;

== matlab function DT4V_System_Model_v17_ref_speed_R2019a/Drive Motor/Electromagnetic Model/Electromagnetic model/Stator flux calculation/MATLAB Function ==
  data: Psi_q_2 input; Psi_tot output; Psi_d_2 input
function Psi_tot = fcn(Psi_q_2, Psi_d_2)
Psi_tot = sqrt(Psi_q_2^2+Psi_d_2^2);
end

== matlab function DT4V_System_Model_v17_ref_speed_R2019a/Power Electronics2/AC//DC Converter/Half-Bridge 3/MATLAB Function ==
  data: Vdc input; Vphase output; Iphase input; VT input; R_0 input; Idc output; Pcond output
function [Vphase, Idc, Pcond] = fcn(Vdc,Iphase,VT,R_0)


%%%%%%%%%%%%%%%%%%%%%%

if Iphase>=0 %&& Vphase1>=0.7 % current from brigde to motor
    Vphase= Vdc+VT+R_0*Iphase;
    Idc=Iphase;
    Pcond_d1= 0;
    Pcond_d2= (VT+R_0*Iphase)*Iphase;
    
else
    Vphase=-VT+R_0*Iphase;
    Idc=0;    
    Pcond_d2= 0;
    Pcond_d1= (-VT+R_0*Iphase)*Iphase;
    
end
Pcond = Pcond_d1+Pcond_d2;

== matlab function DT4V_System_Model_v17_ref_speed_R2019a/Power Electronics2/DC//AC Converter/Half-Bridge 1/MATLAB Function ==
  data: d input; Vdc input; Vphase output; Iphase input; Vce_on input; Rce_on input; Vf_0 input; Rd input; Idc output; Pcond output
function [Vphase, Idc, Pcond] = fcn(d, Vdc,Iphase,  Vce_on, Rce_on,Vf_0,Rd)
td=0;
fs=0;
if d>0 
    theta_u= d-td*fs;
    theta_l=1-d-td*fs;
else
    theta_u= 0;
    theta_l=0;
end
%%%%%%%%%%%%%%%%%%%%%%

if Iphase>0 % current from brigde to motor
    Vphase= theta_u*(Vdc-(Vce_on+Rce_on*Iphase))-(1-theta_u)*(Vf_0+Rd*Iphase);
    Idc=theta_u*Iphase;
    Pcond_s1=theta_u*(Vce_on+Rce_on*Iphase)*Iphase ;
    Pcond_s2=0 ;
    Pcond_d1= 0;
    Pcond_d2= (1-theta_u)*(Vf_0+Rd*Iphase)*Iphase;
    
else
    Vphase= theta_l*(Vce_on-Rce_on*Iphase)+(1-theta_l)*(Vdc+Vf_0-Rd*Iphase);
    Idc=(1-theta_l)*Iphase;    
    Pcond_s1=0 ;
    Pcond_s2=-theta_l*(Vce_on-Rce_on*Iphase)*Iphase;
    Pcond_d1= -(1-theta_l)*(Vf_0-Rd*Iphase)*Iphase;    
    Pcond_d2= 0;
    
end
Pcond = abs(Pcond_s1)+abs(Pcond_s2)+abs(Pcond_d1)+abs(Pcond_d2);

== matlab function DT4V_System_Model_v17_ref_speed_R2019a/Gearbox1/Power loss model/MATLAB Function ==
  data: gear12 input; pair12 input; P_loss output; gear34 input; pair34 input; bear input; oil input; params_identified input; Tin input; Nin input; P_gear output; P_bearing output; P_churning output; P_belt output; T_loss_input output; T_loss_interm output; T_loss_out output; Te_oil input
%%% - Power loss function based on model Sven for integration with Simulink model - %%%
function [P_loss, P_gear, P_bearing, P_churning,P_belt,T_loss_input,T_loss_interm,T_loss_out] = ...
            DT4V_power_loss_update(gear12, pair12, gear34, pair34, bear, oil, params_identified, Tin, Nin,Te_oil)
% =========================================================================
% [P_loss, P_gear, P_bearing, P_churning] = PowerLosses(gear, pair, bear, oil, Tin, Nin)
% =========================================================================
%
% Inputs:
%
%   gear12   = containing geometry of pinion and gear 1-2       [struct]
%   pair12   = containing geometry of gear pair 1-2             [struct]
%   gear34   = containing geometry of pinion and gear 3-4       [struct]
%   pair34   = containing geometry of gear pair 3-4             [struct]
%   bear     = containing bearing data for loss computation     [struct]
%   oil      = containing oil data for loss computation         [struct]
%   Tin      = input shaft torque                               [scalar]
%   Nin      = input shaft rpm                                  [scalar]

TR_tot         = gear12(2).z/gear12(1).z * gear34(2).z/gear34(1).z;
TR_12          = gear12(2).z/gear12(1).z;
fg             = params_identified.fg;

% Te_B_in     = Te_oil;
% Te_B_interm = Te_oil;
% Te_B_out    = Te_oil;
% Te_sump     = Te_oil;

% oil.v_bearing1 = viscosity_temp_curve(oil,Te_B_in);
% oil.v_bearing2 = viscosity_temp_curve(oil,Te_B_interm);
% oil.v_bearing3 = viscosity_temp_curve(oil,Te_B_out);
% oil.v_sump     = viscosity_temp_curve(oil,Te_sump);
% Problem with measured sump temperature, bearing 3 temp used

%%% -  Load-independent (viscous) losses -- %%%
%% Viscous bearing loss + churning loss
[T_bearing_v_tot,bear,T_churning_tot,T_chur_1,T_chur_2,T_chur_3,T_chur_4] = ...
    viscous_losses(Nin,Te_oil,gear12,gear34,bear,oil,params_identified); % Temperature3
T_loss_viscous_tot = T_churning_tot + T_bearing_v_tot;
P_churning         = T_churning_tot*Nin;

%%% -  Load-dependent (friction) losses -- %%%
Nin34       = Nin/(gear12(2).z/gear12(1).z);
Nout        = Nin34 /( gear34(2).z/gear34(1).z);
Tin_0       = Tin - T_chur_1;
Tin_1       = Tin_0;
Tin_2       = Tin_0;
%% - Bearings friction losses input shaft - %
% -> iterating as load-dependent bearing losses depend on and influence the
% load level
counter_b1 = 1;
maxit      = 5;

% run loop already prior to actual loop such that Simulink is happy:
top_contact_in = 1; % contact gear1 is at the top of the shaft
[bear(1).F,bear(2).F,bear(1).Seq,bear(2).Seq,bear(1).Fr,bear(2).Fr,bear(1).Fa,bear(2).Fa] = ...
    bearing_forces_1_gear_on_shaft(gear12,pair12,bear(1),bear(2),abs(Tin_2),top_contact_in);
v12 = viscosity_temp_curve(oil,Te_oil);
[M_rr1,M_sl1,M_drag1,M_seal1,T_B1] = torque_loss_SKF(bear(1),abs(Nin),v12);
[M_rr2,M_sl2,M_drag2,M_seal2,T_B2] = torque_loss_SKF(bear(2),abs(Nin),v12);
Tin_2 = Tin_0-T_B1/1000-T_B2/1000;
diff = abs(Tin_2-Tin_1);
Tin_1 = Tin_2;
counter_b1 = counter_b1+1;

while (diff > 0.001*abs(Tin_2) && counter_b1 <= maxit)
    % (Simplified) force analysis gear-bearing system
    [bear(1).F,bear(2).F,bear(1).Seq,bear(2).Seq,bear(1).Fr,bear(2).Fr,bear(1).Fa,bear(2).Fa] = ...
        bearing_forces_1_gear_on_shaft(gear12,pair12,bear(1),bear(2),abs(Tin_2),top_contact_in);
    
    [M_rr1,M_sl1,M_drag1,M_seal1,T_B1] = torque_loss_SKF(bear(1),abs(Nin),v12);
    [M_rr2,M_sl2,M_drag2,M_seal2,T_B2] = torque_loss_SKF(bear(2),abs(Nin),v12);

    Tin_2 = Tin_0-T_B1/1000-T_B2/1000;
    diff = abs(Tin_2-Tin_1);
    Tin_1 = Tin_2;
    counter_b1 = counter_b1+1;
end

%% - Friction losses gear pair 1 - %
oil.v_sump = viscosity_temp_curve(oil,Te_oil);
P_gear12 = power_loss_tooth_friction(pair12,gear12,oil,abs(Tin_1),Nin);

Tin34 = gear12(2).z/gear12(1).z * Tin_1 - T_chur_2 - T_chur_3 - ...
        fg*P_gear12.*(Nin/60*2*pi).^-1*(gear12(2).z/gear12(1).z);
Tin34_bear = Tin34;
    
%% - Bearing friction losses intermediate shaft - %  
Tin34_bear_save = 0;
counter_b2 = 1;          %counting how many iterations
% - prior to loop run variables such that Simulink is happy:
top_contact_in1 = -1; % contact gear2 is at the bottom of the shaft
top_contact_in2 = 1; % contact gear3 is at the top of the shaft
[bear(3).F,bear(4).F,bear(3).Seq,bear(4).Seq,bear(3).Fr,bear(4).Fr,bear(3).Fa,bear(4).Fa] = ...
    bearing_forces_2_gears_on_shaft(gear12,pair12,gear34,pair34,...
    bear(3),bear(4),abs(Tin_1),abs(Tin34_bear),top_contact_in1,top_contact_in2);
v34 = viscosity_temp_curve(oil,Te_oil);
[M_rr3,M_sl3,M_drag3,M_seal3,T_B3] = torque_loss_SKF(bear(3),abs(Nin34),v34);
[M_rr4,M_sl4,M_drag4,M_seal4,T_B4] = torque_loss_SKF(bear(4),abs(Nin34),v34);
Tin34_bear = Tin34 - T_B3/1000 - T_B4/1000;
diff = abs(Tin34_bear-Tin34_bear_save);
Tin34_bear_save = Tin34_bear;
counter_b2 = counter_b2+1;
while diff > 0.001*abs(Tin34_bear) && counter_b2 <= maxit
    [bear(3).F,bear(4).F,bear(3).Seq,bear(4).Seq,bear(3).Fr,bear(4).Fr,bear(3).Fa,bear(4).Fa] = ...
        bearing_forces_2_gears_on_shaft(gear12,pair12,gear34,pair34,...
        bear(3),bear(4),abs(Tin_1),abs(Tin34_bear),top_contact_in1,top_contact_in2);
    
    [M_rr3,M_sl3,M_drag3,M_seal3,T_B3] = torque_loss_SKF(bear(3),abs(Nin34),v34);
    [M_rr4,M_sl4,M_drag4,M_seal4,T_B4] = torque_loss_SKF(bear(4),abs(Nin34),v34);

    Tin34_bear = Tin34 - T_B3/1000 - T_B4/1000;

    diff = abs(Tin34_bear-Tin34_bear_save);
    Tin34_bear_save = Tin34_bear;

    counter_b2 = counter_b2+1;
end

Tin34 = Tin34_bear;

%% gear power loss second pair
P_gear34 = power_loss_tooth_friction(pair34,gear34,oil,abs(Tin34),abs(Nin34));
P_gear = fg*(P_gear12+P_gear34);
T_gear = P_gear.*(Nin/60*2*pi).^-1;

%% Bearing forces output shaft
Tout        = Tin34*(gear34(2).z/gear34(1).z) - T_chur_4*...
              ((gear12(2).z/gear12(1).z)*(gear34(2).z/gear34(1).z)) - ...
              fg*P_gear34.*(Nin34/60*2*pi).^-1*(gear34(2).z/gear34(1).z);
Tout_bear   = Tout;
Tout_bear_save = 0;
counter_b3 = 1;

%% Let Simulink be :)))
top_contact_out = -1; % contact gear4 is at the bottom of the shaft
Dpulley = 0.299;    % diameter of the pulley on the output shaft on which the belt is attached (in m)
[bear(5).F,bear(6).F,bear(5).Seq,bear(6).Seq,bear(5).Fr,bear(6).Fr,bear(5).Fa,bear(6).Fa] =...
    bearing_forces_1_gear_on_shaft_and_belt(gear34,pair34,bear(5),bear(6),abs(Tin34),top_contact_out,Tout_bear,Dpulley);        
v56 = viscosity_temp_curve(oil,Te_oil);
[M_rr5,M_sl5,M_drag5,M_seal5,T_B5] = torque_loss_SKF(bear(5),abs(Nout),v56);
[M_rr6,M_sl6,M_drag6,M_seal6,T_B6] = torque_loss_SKF(bear(6),abs(Nout),v56);

Tout_bear = Tout - T_B5/1000 - T_B6/1000;
diff = abs(Tout_bear- Tout_bear_save);
Tout_bear_save = Tout_bear;
counter_b3 = counter_b3 +1;
while diff > 0.001*abs(Tout_bear) && counter_b3 <= maxit
    [bear(5).F,bear(6).F,bear(5).Seq,bear(6).Seq,bear(5).Fr,bear(6).Fr,bear(5).Fa,bear(6).Fa] =...
        bearing_forces_1_gear_on_shaft_and_belt(gear34,pair34,bear(5),bear(6),abs(Tin34),top_contact_out,Tout_bear,Dpulley);        
    
    [M_rr5,M_sl5,M_drag5,M_seal5,T_B5] = torque_loss_SKF(bear(5),abs(Nout),v56);
    [M_rr6,M_sl6,M_drag6,M_seal6,T_B6] = torque_loss_SKF(bear(6),abs(Nout),v56);

    Tout_bear = Tout - T_B5/1000 - T_B6/1000;
    diff = abs(Tout_bear- Tout_bear_save);
    Tout_bear_save = Tout_bear;

    counter_b3 = counter_b3 +1;
end

% cte_est_load   = params_identified.cte_est_load;
% Tout = Tout_bear-cte_est_load*TR_tot;

%% Summing losses to total contributions
T_rr_total   = (M_rr1 + M_rr2 + (M_rr3+M_rr4)/TR_12 + (M_rr5+M_rr6)/TR_tot) / 1000;
T_sl_total   = (M_sl1 + M_sl2 + (M_sl3+M_sl4)/TR_12 + (M_sl5+M_sl6)/TR_tot) / 1000;
T_drag_total = (M_drag1 + M_drag2 + (M_drag3+M_drag4)/TR_12 + (M_drag5+M_drag6)/TR_tot) / 1000;
T_seal_total = (M_seal1 + M_seal2 + (M_seal3+M_seal4)/TR_12 + (M_seal5+M_seal6)/TR_tot) / 1000;

T_bearing_F_tot = T_rr_total + T_sl_total + T_drag_total + T_seal_total;
T_bearing       = T_bearing_F_tot + T_bearing_v_tot;
P_bearing       = T_bearing * Nin*2*pi/60;

belteff = beltmap((Tin-fg*T_gear-T_bearing_F_tot-T_loss_viscous_tot)*TR_tot,Nout);
T_belt = (1-belteff).*Tin;
P_belt = T_belt * Nout*2*pi/60;
%     T_loss_tot  = Tq_in-abs(Tq_out_est_filt_GB);
T_bearings_input    = (M_rr1 + M_rr2 + M_sl1 + M_sl2 + M_drag1 + M_drag2 + M_seal1 + M_seal2)/1000 + ...
                      bear(1).T_loss_v + bear(2).T_loss_v;
T_bearings_interm   = (M_rr3 + M_rr4 + M_sl3 + M_sl4 + M_drag3 + M_drag4 + M_seal3 + M_seal4)/1000 + ...
                      bear(3).T_loss_v + bear(4).T_loss_v;
T_bearings_out      = (M_rr5 + M_rr6 + M_sl5 + M_sl6 + M_drag5 + M_drag6 + M_seal5 + M_seal6)/1000 + ...
                      bear(5).T_loss_v + bear(6).T_loss_v;
T_gears_input       = T_chur_1;
T_gears_interm      = T_chur_2 + T_chur_3 + P_gear12/(Nin34*2*pi/60);
T_gears_out         = T_chur_4 + P_gear34/(Nout*2*pi/60);
T_loss_input        = T_gears_input  + T_bearings_input;
T_loss_interm       = T_gears_interm + T_bearings_interm;
T_loss_out          = T_gears_out    + T_bearings_out;

P_loss      = P_gear + P_churning + P_bearing + P_belt;
